simulink model "Mass1_sim"  (R2024a)
settings: Solver=VariableStepAuto  StartTime=0.0  StopTime=sim_time  RelTol=1e-3
undefined symbols (not defined in the file): b, F, k, m
settings Model: Creator=alisr_qxy0y9  LastModifiedBy=alisr_qxy0y9

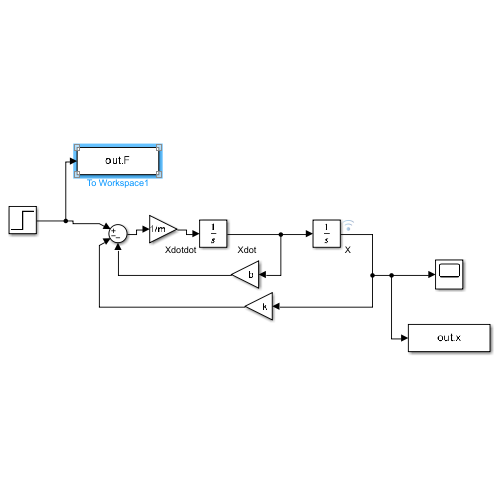
[thumbnail: Simulink's stored preview of the top-level diagram]
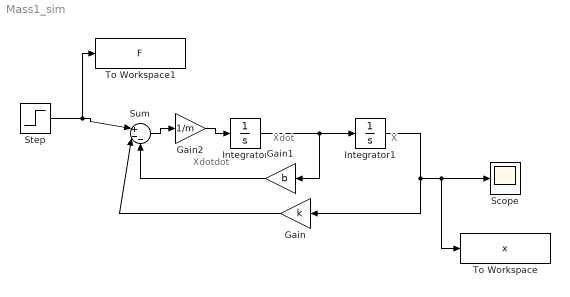
== system Mass1_sim ==
  note: Xdotdot
  note: Xdot
  note: X
  Gain : Gain  Gain=k
  Gain1 : Gain  Gain=b
  Gain2 : Gain  Gain=1/m
  Integrator : Integrator
  Integrator1 : Integrator
  Scope : Scope
  Step : Step  After=F  SampleTime=0
  Sum : Sum  Inputs=|+--
  To Workspace : ToWorkspace  VariableName=x  SaveFormat=Timeseries  SampleTime=-1
  To Workspace1 : ToWorkspace  VariableName=F  SaveFormat=Timeseries  SampleTime=-1
  wires:
  Integrator/1 -> Gain1/1, Integrator1/1
  Integrator1/1 -> To Workspace/1, Scope/1, Gain/1
  Step/1 -> To Workspace1/1, Sum/1
  Gain1/1 -> Sum/3
  Gain/1 -> Sum/2
  Sum/1 -> Gain2/1
  Gain2/1 -> Integrator/1
